simulink model "Studio4"  (R2017b)
settings: Solver=ode45  StartTime=0.  StopTime=16  FixedStep=0.2  MaxStep=0.05  RelTol=1e-8  AbsTol=1e-8  EnableMultiTasking=on
settings Model: ExtModeTrigMode=oneshot  ExtModeArmWhenConnect=off  Creator=LEVIENKL  LastModifiedBy=carlislt
settings DataIOCC: SaveFormat=Array  SignalLoggingSaveFormat=ModelDataLogs  SaveOutput=off  SaveTime=off  SignalLoggingName=sigsOut
settings OptimizationCC: BlockReduction=off  BooleanDataType=off  ExpressionDepthLimit=2147483647  InitFltsAndDblsToZero=on  LifeSpan=inf
settings DebuggingCC: SaveWithParameterizedLinksMsg=none  UnderspecifiedInitializationDetection=Classic  MergeDetectMultiDrivingBlocksExec=none  SignalResolutionControl=TryResolveAllWithWarning  MultiTaskDSMMsg=warning  MultiTaskCondExecSysMsg=none  FcnCallInpInsideContextMsg=warning  AllowSymbolicDim=off  StateNameClashWarn=warning  SFUnexpectedBacktrackingDiag=warning  SFNoUnconditionalDefaultTransitionDiag=warning  SFExecutionAtInitializationDiag=none
settings HardwareCC: ProdBitPerPointer=32  ProdBitPerSizeT=32  ProdBitPerPtrDiffT=32  ProdLargestAtomicFloat=None  ProdIntDivRoundTo=Undefined  ProdEndianess=Unspecified  ProdWordSize=32  ProdHWDeviceType=32-bit Generic  TargetUnknown=on
settings ModelReferenceCC: PropagateSignalLabelsOutOfModel=off
settings CodeAppCC: StateflowObjectComments=on
settings GRTTargetCC: TargetFcnLib=ansi_tfl_tmw.mat  TargetLangStandard=C89/C90 (ANSI)  GeneratePreprocessorConditionals=Disable all  CombineOutputUpdateFcns=off  GRTInterface=on
settings ConfigComp: CovMetricSettings=dw  CovHtmlReporting=on  CovSaveCumulativeToWorkspaceVar=on  CovSaveSingleToWorkspaceVar=on  CovExternalEMLEnable=off  CovSFcnEnable=off

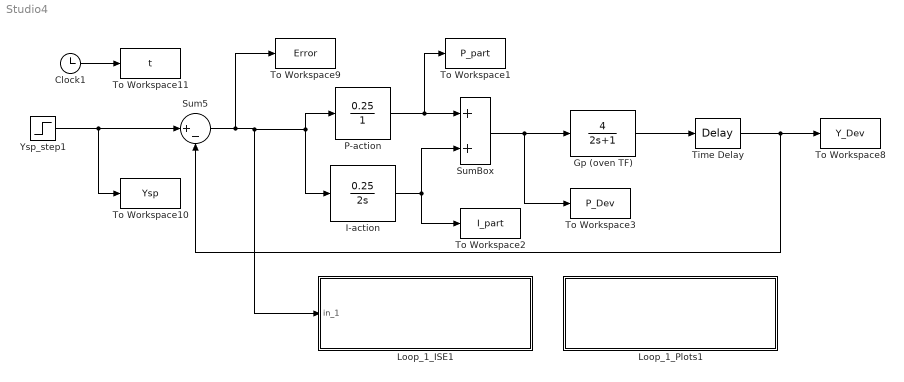
== system Studio4 ==
  Clock1 : Clock
  Gp (oven TF) : TransferFcn  Numerator=[4]  Denominator=[2 1]
  I-action : TransferFcn  Numerator=[0.25]  Denominator=[2 0]
  Loop_1_ISE1 : Subsystem  mask(Integral Squarred Evaluation - Loop 1){}
      settings: OpenFcn=ISE1
      mask Help: This block calculates and plots loop #1 ISE.
      mask Display: disp('After Loop 1 Simulation:\n Double Click for ISE evaluation\n (uses ISE1.p)')
  Loop_1_Plots1 : Subsystem  mask(Y,U,E Plots - Loop 1){}
      settings: OpenFcn=YPEplots
      mask Help: This block loop #1 Y,U,Error in 3x1 Figure Window.
      mask Display: disp('After Loop 1 Simulation:\n Double Click for Y, P, Error Plots\n (uses YPEplots.p)')
  "P-action " : TransferFcn  Numerator=[0.25]  Denominator=[0 1]
  Sum5 : Sum  Inputs=|+-  SaturateOnIntegerOverflow=on  InputSameDT=on  OutDataTypeStr=Inherit: Same as first input
  SumBox : Sum
  Time Delay : TransportDelay  DelayTime=0
      settings: AttributesFormatString=Delay=%<DelayTime>
  To Workspace1 : ToWorkspace  VariableName=P_part  SampleTime=-1
  To Workspace10 : ToWorkspace  VariableName=Ysp  SampleTime=-1
  To Workspace11 : ToWorkspace  VariableName=t  SampleTime=-1
  To Workspace2 : ToWorkspace  VariableName=I_part  SampleTime=-1
  To Workspace3 : ToWorkspace  VariableName=P_Dev  SampleTime=-1
  To Workspace8 : ToWorkspace  VariableName=Y_Dev  SampleTime=-1
  To Workspace9 : ToWorkspace  VariableName=Error  SampleTime=-1
  Ysp_step1 : Step  Time=2  After=10  SampleTime=0
      settings: AttributesFormatString=%<Before> to %<After>\nat %<Time>
  wires:
  Clock1/1 -> To Workspace11/1
  Ysp_step1/1 -> To Workspace10/1, Sum5/1
  Sum5/1 -> To Workspace9/1, "P-action "/1, I-action/1, Loop_1_ISE1/1(in_1)
  "P-action "/1 -> To Workspace1/1, SumBox/1
  I-action/1 -> To Workspace2/1, SumBox/2
  SumBox/1 -> Gp (oven TF)/1, To Workspace3/1
  Gp (oven TF)/1 -> Time Delay/1
  Time Delay/1 -> Sum5/2, To Workspace8/1

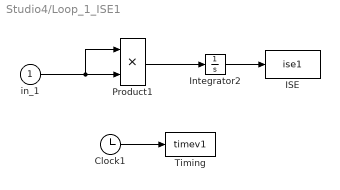
== system Studio4/Loop_1_ISE1 ==
  in_1 : Inport
  Clock1 : Clock
  ISE : ToWorkspace  VariableName=ise1
      settings: MaxDataPoints=20000
  Integrator2 : Integrator
  Product1 : Product  SaturateOnIntegerOverflow=on  RndMeth=Zero  InputSameDT=on  OutDataTypeStr=Inherit: Same as first input
  Timing : ToWorkspace  VariableName=timev1
      settings: MaxDataPoints=20000
  wires:
  in_1/1 -> Product1/2, Product1/1
  Integrator2/1 -> ISE/1
  Clock1/1 -> Timing/1
  Product1/1 -> Integrator2/1

== system Studio4/Loop_1_Plots1 ==
